simulink library "pasp_lib"  (Simulink 7.3)
settings: Solver=ode45  StartTime=0.0  StopTime=10.0  RelTol=1e-3
libraries: xps_library x16, xbsIndex_r4 x7
settings Model: Creator=tfiliba  LastModifiedBy=tfiliba

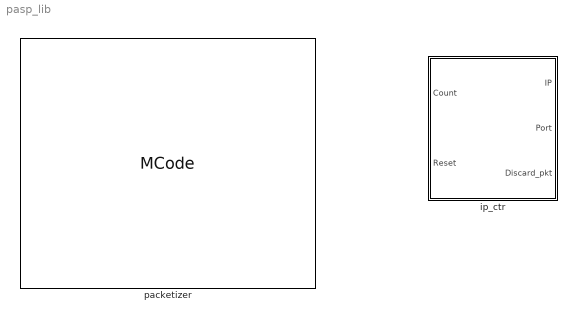
== system pasp_lib ==
  ip_ctr : Subsystem  mask(ip_ctr){numcomputers=8}
      mask prompts: numcomputers "Num IPs (Must be power of 2)"
      mask init:
      | ip_ctr_init(gcb,...
      |     'numcomputers',numcomputers)
      settings: AttributesFormatString=IPs=8
  packetizer : xbsIndex_r4/MCode  mfname=packetizer  explicit_period=off  period=1  inputsTable={'boundInpExpr'=>['','','','','','',''],'inputs'=>['sync','din','sys_counter','packet_size','numcomputers','numtengbe','tengbe_id']}  outputsTable={'outputs'=>['dout','valid','end_of_frame','st'],'suppressOut'=>['off','off','off','on']}  dbl_ovrd=off  enable_stdout=off  enable_debug=off  suppress_output=on  defparams={}  hide_port_list={'st'}  block_type=mcode
      settings: block_version=11.4

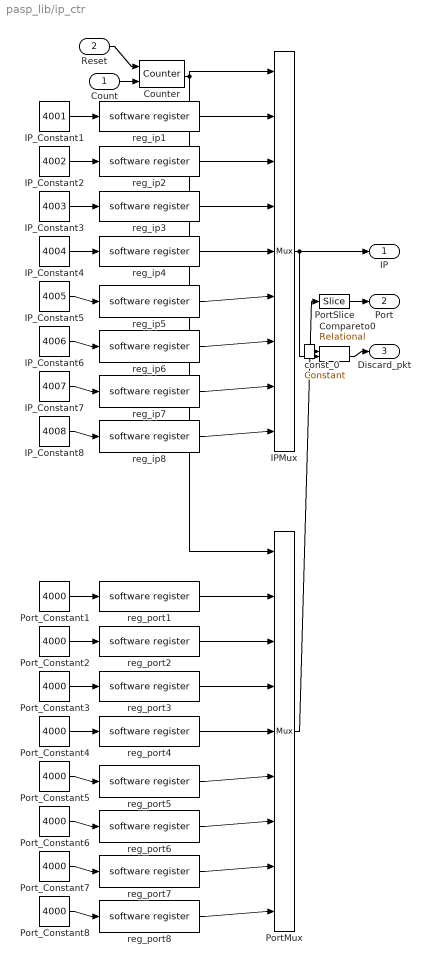
== system pasp_lib/ip_ctr ==
  Count : Inport
  Reset : Inport  Port=2  OutDataType=sfix(16)  OutScaling=2^0
  Compareto0 : xbsIndex_r4/Relational  mode=a=b  en=off  latency=1  dbl_ovrd=off  block_type=relational
  Counter : xbsIndex_r4/Counter  cnt_type=Free Running  cnt_to=Inf  operation=Up  start_count=0  cnt_by_val=1  arith_type=Unsigned  n_bits=3  bin_pt=0  load_pin=off  rst=on  en=on  explicit_period=on  period=1  dbl_ovrd=off  use_behavioral_HDL=off  implementation=Fabric  block_type=counter
      settings: block_version=11.4
  IPMux : xbsIndex_r4/Mux  inputs=8  en=off  latency=3  precision=Full  arith_type=Unsigned  n_bits=16  bin_pt=14  quantization=Truncate  overflow=Wrap  dbl_ovrd=off  block_type=mux
      settings: block_version=11.4
  IP_Constant1 : Constant  Value=4001  OutDataType=sfix(16)  OutScaling=2^0
  IP_Constant2 : Constant  Value=4002  OutDataType=sfix(16)  OutScaling=2^0
  IP_Constant3 : Constant  Value=4003  OutDataType=sfix(16)  OutScaling=2^0
  IP_Constant4 : Constant  Value=4004  OutDataType=sfix(16)  OutScaling=2^0
  IP_Constant5 : Constant  Value=4005  OutDataType=fixdt(1, 16)  OutScaling=2^0
  IP_Constant6 : Constant  Value=4006  OutDataType=fixdt(1, 16)  OutScaling=2^0
  IP_Constant7 : Constant  Value=4007  OutDataType=fixdt(1, 16)  OutScaling=2^0
  IP_Constant8 : Constant  Value=4008  OutDataType=fixdt(1, 16)  OutScaling=2^0
  PortMux : xbsIndex_r4/Mux  inputs=8  en=off  latency=3  precision=Full  arith_type=Unsigned  n_bits=16  bin_pt=14  quantization=Truncate  overflow=Wrap  dbl_ovrd=off  block_type=mux
      settings: block_version=11.4
  PortSlice : xbsIndex_r4/Slice  nbits=16  boolean_output=off  mode=Lower Bit Location + Width  bit1=0  base1=MSB of Input  bit0=0  base0=LSB of Input  dbl_ovrd=off  block_type=slice
  Port_Constant{1..4} (4 alike) : Constant  Value=4000  OutDataType=sfix(16)  OutScaling=2^0
  Port_Constant{5..8} (4 alike) : Constant  Value=4000  OutDataType=fixdt(1, 16)  OutScaling=2^0
  const_0 : xbsIndex_r4/Constant  arith_type=Unsigned  const=0  n_bits=32  bin_pt=0  explicit_period=off  period=1  equ=P=C  opselect=C  inp2=PCIN>>17  opr=+  inp1=P  carry=CIN  dbl_ovrd=off  block_type=constant
      settings: block_version=11.4
  reg_ip1 : xps_library/software register  Tag=xps:sw_reg  SystemSampleTime=-1  io_dir=From Processor  arith_type=Unsigned  bitwidth=32  bin_pt=0  sample_period=1  gw_name=packetizer_dist_gbe_test_dist_gbe_ip_ctr_reg_ip1_user_data_out
      link override pasp_16i16c128s_pasp_dist_gbe_ip_ctr_reg_ip1_user_data_out: arith_type=Unsigned  n_bits=32  bin_pt=0  period=1
  reg_ip2 : xps_library/software register  Tag=xps:sw_reg  SystemSampleTime=-1  io_dir=From Processor  arith_type=Unsigned  bitwidth=32  bin_pt=0  sample_period=1  gw_name=packetizer_dist_gbe_test_dist_gbe_ip_ctr_reg_ip2_user_data_out
      link override pasp_16i16c128s_pasp_dist_gbe_ip_ctr_reg_ip2_user_data_out: arith_type=Unsigned  n_bits=32  bin_pt=0  period=1
  reg_ip3 : xps_library/software register  Tag=xps:sw_reg  SystemSampleTime=-1  io_dir=From Processor  arith_type=Unsigned  bitwidth=32  bin_pt=0  sample_period=1  gw_name=packetizer_dist_gbe_test_dist_gbe_ip_ctr_reg_ip3_user_data_out
      link override pasp_16i16c128s_pasp_dist_gbe_ip_ctr_reg_ip3_user_data_out: arith_type=Unsigned  n_bits=32  bin_pt=0  period=1
  reg_ip4 : xps_library/software register  Tag=xps:sw_reg  SystemSampleTime=-1  io_dir=From Processor  arith_type=Unsigned  bitwidth=32  bin_pt=0  sample_period=1  gw_name=packetizer_dist_gbe_test_dist_gbe_ip_ctr_reg_ip4_user_data_out
      link override pasp_16i16c128s_pasp_dist_gbe_ip_ctr_reg_ip4_user_data_out: arith_type=Unsigned  n_bits=32  bin_pt=0  period=1
  reg_ip5 : xps_library/software register  Tag=xps:sw_reg  SystemSampleTime=-1  io_dir=From Processor  arith_type=Unsigned  bitwidth=32  bin_pt=0  sample_period=1  gw_name=packetizer_dist_gbe_test_dist_gbe_ip_ctr_reg_ip5_user_data_out
  reg_ip6 : xps_library/software register  Tag=xps:sw_reg  SystemSampleTime=-1  io_dir=From Processor  arith_type=Unsigned  bitwidth=32  bin_pt=0  sample_period=1  gw_name=packetizer_dist_gbe_test_dist_gbe_ip_ctr_reg_ip6_user_data_out
  reg_ip7 : xps_library/software register  Tag=xps:sw_reg  SystemSampleTime=-1  io_dir=From Processor  arith_type=Unsigned  bitwidth=32  bin_pt=0  sample_period=1  gw_name=packetizer_dist_gbe_test_dist_gbe_ip_ctr_reg_ip7_user_data_out
  reg_ip8 : xps_library/software register  Tag=xps:sw_reg  SystemSampleTime=-1  io_dir=From Processor  arith_type=Unsigned  bitwidth=32  bin_pt=0  sample_period=1  gw_name=packetizer_dist_gbe_test_dist_gbe_ip_ctr_reg_ip8_user_data_out
  reg_port1 : xps_library/software register  Tag=xps:sw_reg  SystemSampleTime=-1  io_dir=From Processor  arith_type=Unsigned  bitwidth=32  bin_pt=0  sample_period=1  gw_name=packetizer_dist_gbe_test_dist_gbe_ip_ctr_reg_port1_user_data_out
      link override pasp_16i16c128s_pasp_dist_gbe_ip_ctr_reg_port1_user_data_out: arith_type=Unsigned  n_bits=32  bin_pt=0  period=1
  reg_port2 : xps_library/software register  Tag=xps:sw_reg  SystemSampleTime=-1  io_dir=From Processor  arith_type=Unsigned  bitwidth=32  bin_pt=0  sample_period=1  gw_name=packetizer_dist_gbe_test_dist_gbe_ip_ctr_reg_port2_user_data_out
      link override pasp_16i16c128s_pasp_dist_gbe_ip_ctr_reg_port2_user_data_out: arith_type=Unsigned  n_bits=32  bin_pt=0  period=1
  reg_port3 : xps_library/software register  Tag=xps:sw_reg  SystemSampleTime=-1  io_dir=From Processor  arith_type=Unsigned  bitwidth=32  bin_pt=0  sample_period=1  gw_name=packetizer_dist_gbe_test_dist_gbe_ip_ctr_reg_port3_user_data_out
      link override pasp_16i16c128s_pasp_dist_gbe_ip_ctr_reg_port3_user_data_out: arith_type=Unsigned  n_bits=32  bin_pt=0  period=1
  reg_port4 : xps_library/software register  Tag=xps:sw_reg  SystemSampleTime=-1  io_dir=From Processor  arith_type=Unsigned  bitwidth=32  bin_pt=0  sample_period=1  gw_name=packetizer_dist_gbe_test_dist_gbe_ip_ctr_reg_port4_user_data_out
      link override pasp_16i16c128s_pasp_dist_gbe_ip_ctr_reg_port4_user_data_out: arith_type=Unsigned  n_bits=32  bin_pt=0  period=1
  reg_port5 : xps_library/software register  Tag=xps:sw_reg  SystemSampleTime=-1  io_dir=From Processor  arith_type=Unsigned  bitwidth=32  bin_pt=0  sample_period=1  gw_name=packetizer_dist_gbe_test_dist_gbe_ip_ctr_reg_port5_user_data_out
  reg_port6 : xps_library/software register  Tag=xps:sw_reg  SystemSampleTime=-1  io_dir=From Processor  arith_type=Unsigned  bitwidth=32  bin_pt=0  sample_period=1  gw_name=packetizer_dist_gbe_test_dist_gbe_ip_ctr_reg_port6_user_data_out
  reg_port7 : xps_library/software register  Tag=xps:sw_reg  SystemSampleTime=-1  io_dir=From Processor  arith_type=Unsigned  bitwidth=32  bin_pt=0  sample_period=1  gw_name=packetizer_dist_gbe_test_dist_gbe_ip_ctr_reg_port7_user_data_out
  reg_port8 : xps_library/software register  Tag=xps:sw_reg  SystemSampleTime=-1  io_dir=From Processor  arith_type=Unsigned  bitwidth=32  bin_pt=0  sample_period=1  gw_name=packetizer_dist_gbe_test_dist_gbe_ip_ctr_reg_port8_user_data_out
  IP : Outport
  Port : Outport  Port=2
  Discard_pkt : Outport  Port=3
  wires:
  reg_port8/1 -> PortMux/9
  Port_Constant8/1 -> reg_port8/1
  reg_ip8/1 -> IPMux/9
  IP_Constant8/1 -> reg_ip8/1
  reg_port7/1 -> PortMux/8
  Port_Constant7/1 -> reg_port7/1
  reg_ip7/1 -> IPMux/8
  IP_Constant7/1 -> reg_ip7/1
  reg_port6/1 -> PortMux/7
  Port_Constant6/1 -> reg_port6/1
  reg_ip6/1 -> IPMux/7
  IP_Constant6/1 -> reg_ip6/1
  reg_port5/1 -> PortMux/6
  Port_Constant5/1 -> reg_port5/1
  reg_ip5/1 -> IPMux/6
  IP_Constant5/1 -> reg_ip5/1
  reg_port4/1 -> PortMux/5
  Port_Constant4/1 -> reg_port4/1
  reg_ip4/1 -> IPMux/5
  IP_Constant4/1 -> reg_ip4/1
  reg_port3/1 -> PortMux/4
  Port_Constant3/1 -> reg_port3/1
  reg_ip3/1 -> IPMux/4
  IP_Constant3/1 -> reg_ip3/1
  reg_port2/1 -> PortMux/3
  Port_Constant2/1 -> reg_port2/1
  reg_ip2/1 -> IPMux/3
  IP_Constant2/1 -> reg_ip2/1
  reg_port1/1 -> PortMux/2
  Port_Constant1/1 -> reg_port1/1
  reg_ip1/1 -> IPMux/2
  IP_Constant1/1 -> reg_ip1/1
  Compareto0/1 -> Discard_pkt/1
  const_0/1 -> Compareto0/1
  PortSlice/1 -> Port/1
  PortMux/1 -> PortSlice/1
  IPMux/1 -> Compareto0/2, IP/1
  Counter/1 -> PortMux/1, IPMux/1
  Count/1 -> Counter/2
  Reset/1 -> Counter/1
